simulink subsystem "Reefscape_Sensor_Processing_sub"  (R2023b)
settings: Solver=VariableStepAuto  StartTime=0.0  StopTime=10.0  RelTol=1e-3
undefined symbols (not defined in the file): Elevator_Height_PickupLower_Reset, Elevator_Height_Top_Reset, Elevator_MotorRev_to_Inch
libraries: simulink x3
settings Model: Creator=ander  LastModifiedBy=ander

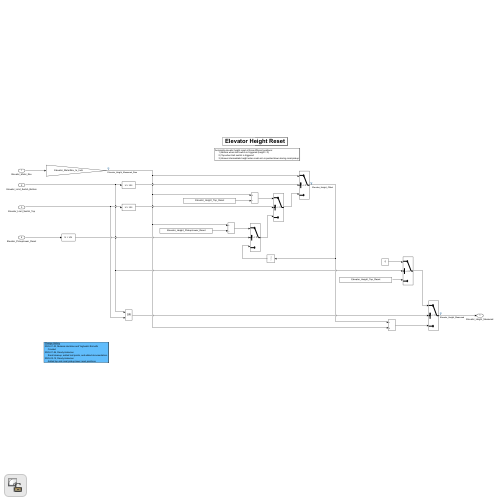
[thumbnail: Simulink's stored preview of the top-level diagram]
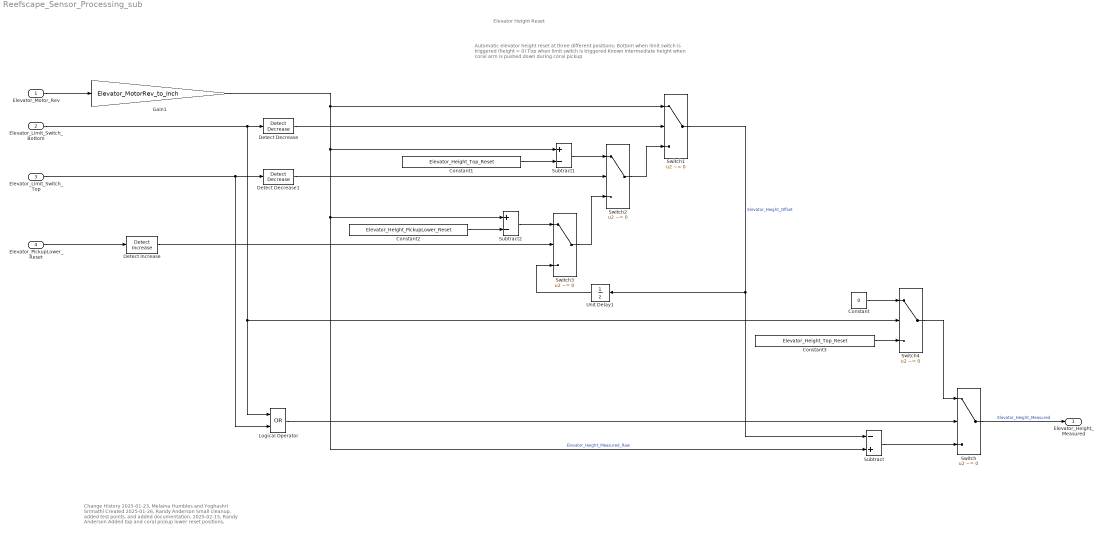
== system Reefscape_Sensor_Processing_sub ==
  note: Change History
      | 2025-01-23, Melaina Humbles and Yoghashri Srimathi
      | Created
      | 2025-01-26, Randy Anderson
      | Small cleanup, added test points, and added documentation.
      | 2025-02-15, Randy Anderson
      | Added top and coral pickup lower reset positions.
  note: Elevator Height Reset
  note: Automatic elevator height reset at three different positions:
      | Bottom when limit switch is triggered (height = 0)
      | Top when limit switch is triggered
      | Known intermediate height when coral arm is pushed down during coral pickup
  Elevator_Motor_Rev : Inport
  Elevator_Limit_Switch_Bottom : Inport  Port=2
  Elevator_Limit_Switch_Top : Inport  Port=3
  Elevator_PickupLower_Reset : Inport  Port=4
  Constant : Constant  Value=0
  Constant1 : Constant  Value=Elevator_Height_Top_Reset
  Constant2 : Constant  Value=Elevator_Height_PickupLower_Reset
  Constant3 : Constant  Value=Elevator_Height_Top_Reset
  Detect Decrease : simulink/Logic and Bit Operations/Detect Decrease  vinit=0.0  OutDataTypeStr=boolean
  Detect Decrease1 : simulink/Logic and Bit Operations/Detect Decrease  vinit=0.0  OutDataTypeStr=boolean
  Detect Increase : simulink/Logic and Bit Operations/Detect Increase  vinit=0.0  OutDataTypeStr=boolean
  Gain1 : Gain  Gain=Elevator_MotorRev_to_Inch
  Logical Operator : Logic  Operator=OR  AllPortsSameDT=off  OutDataTypeStr=boolean
  Subtract : Sum  Inputs=-+
  Subtract1 : Sum  Inputs=+-
  Subtract2 : Sum  Inputs=+-
  Switch{,1..4} (5 alike) : Switch  Criteria=u2 ~= 0  SaturateOnIntegerOverflow=off  InputSameDT=off
  Unit Delay1 : UnitDelay  SampleTime=-1  HasFrameUpgradeWarning=on
  Elevator_Height_Measured : Outport
  wires:
  Detect Increase/1 -> Switch3/2
  Elevator_PickupLower_Reset/1 -> Detect Increase/1
  Logical Operator/1 -> Switch/2
  Switch4/1 -> Switch/1
  Constant3/1 -> Switch4/3
  Constant/1 -> Switch4/1
  Unit Delay1/1 -> Switch3/3
  Switch3/1 -> Switch2/3
  Subtract2/1 -> Switch3/1
  Constant2/1 -> Subtract2/2
  Constant1/1 -> Subtract1/2
  Subtract1/1 -> Switch2/1
  Elevator_Limit_Switch_Top/1 -> Logical Operator/2, Detect Decrease1/1
  Detect Decrease1/1 -> Switch2/2
  Switch2/1 -> Switch1/3
  Gain1/1 -> Subtract2/1, Subtract/2, Subtract1/1, Switch1/1  "Elevator_Height_Measured_Raw"
  Subtract/1 -> Switch/3
  Switch/1 -> Elevator_Height_Measured/1  "Elevator_Height_Measured"
  Switch1/1 -> Subtract/1, Unit Delay1/1  "Elevator_Height_Offset"
  Detect Decrease/1 -> Switch1/2
  Elevator_Motor_Rev/1 -> Gain1/1
  Elevator_Limit_Switch_Bottom/1 -> Logical Operator/1, Switch4/2, Detect Decrease/1
